simulink model "Pendulum_Noise"  (R2016b)
settings: Solver=VariableStepAuto  StartTime=0.0  StopTime=15  RelTol=1e-3
values from neighbouring files (symbols this model uses):
  A = [0 1; -g/l 0]    [Pendulum.m]
  B = [0; tau/m/l^2]    [Pendulum.m]
  C = [1 0]    [Pendulum.m]
  D = 0    [Pendulum.m]
  g = 9.81    [Pendulum.m]
  l = 1    [Pendulum.m]
  m = 1    [Pendulum.m]
  tau = 1    [Pendulum.m]
undefined symbols (not defined in the file or in its folder): Continuous, Time
libraries: simulink x1, ctrlSharedLib x1
settings Model: Creator=Daniel  LastModifiedBy=Daniel

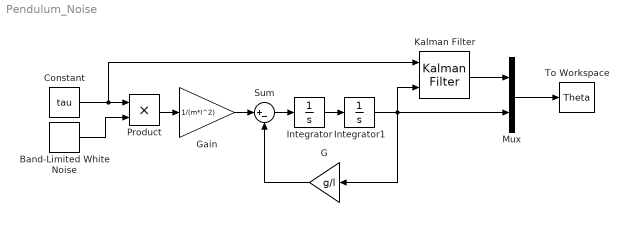
== system Pendulum_Noise ==
  Band-Limited White Noise : simulink/Sources/Band-Limited White Noise  Cov=[0.01]  Ts=0.01  seed=[23341]
  Constant : Constant  Value=tau
  G : Gain  Gain=g/l
  Gain : Gain  Gain=1/(m*l^2)
  Integrator : Integrator
  Integrator1 : Integrator
  Kalman Filter : ctrlSharedLib/Kalman Filter  TimeDomain=Continuous-Time  UseCurrentEstimator=on  ModelSource=Individual A, B, C, D matrices  ModelSourceVariable=ss(0.95,1,1,0,1)  A=A  B=B  C=C  D=D  NumberOfStates=1  NumberOfInputs=1  NumberOfOutputs=1  InitialEstimateSource=Dialog  X0=[0.2 0]  P0=10  UseK=off  UseGH=off  NumberOfProcessNoiseInputs=1  G=1  TimeInvariantG=on  H=0  TimeInvariantH=on  Q=0.05  TimeInvariantQ=on  R=1  TimeInvariantR=on  N=0  TimeInvariantN=on  AddInputPort=on  AddEnablePort=off  OutputEstimatedY=off  OutputP=off  Ts=-1
  Mux : Mux  Inputs=2
  Product : Product
  Sum : Sum  Inputs=|+-
  To Workspace : ToWorkspace  VariableName=Theta  SaveFormat=Timeseries  SampleTime=-1
  wires:
  Product/1 -> Gain/1
  Gain/1 -> Sum/1
  Integrator/1 -> Integrator1/1
  Sum/1 -> Integrator/1
  G/1 -> Sum/2
  Band-Limited White Noise/1 -> Product/2
  Constant/1 -> Kalman Filter/1, Product/1
  Integrator1/1 -> Mux/2, Kalman Filter/2, G/1
  Kalman Filter/1 -> Mux/1
  Mux/1 -> To Workspace/1
